simulink model "snb_bc"  (R2012b)
settings: Solver=FixedStepDiscrete  SolverMode=SingleTasking  StartTime=0.0  StopTime=10000  RelTol=1e-3
undefined symbols (not defined in the file): Down, pfb_coeff_gen_calc, Up
libraries: xbsIndex_r4 x19640, casper_library_misc x44, casper_library_delays x18, casper_library_communications x8, xps_library x3
(part 103 of 163)

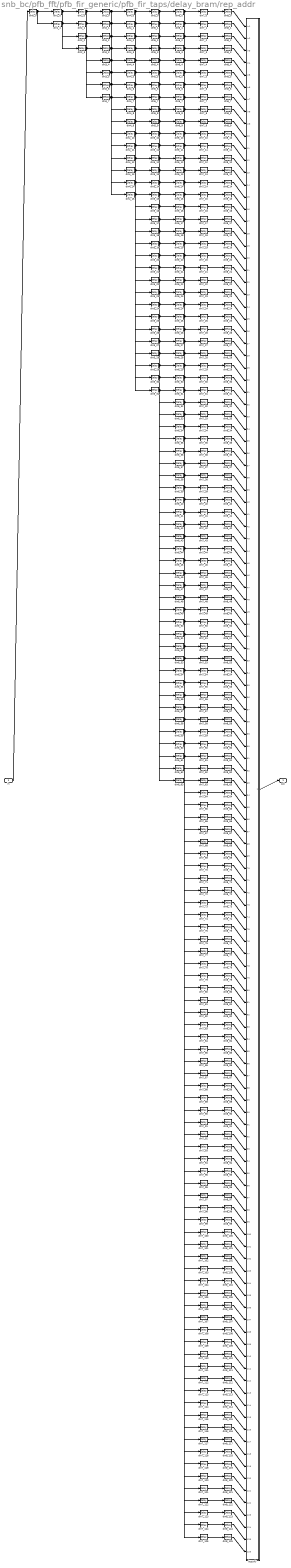
== system snb_bc/pfb_fft/pfb_fir_generic/pfb_fir_taps/delay_bram/rep_addr ==
  in : Inport
  bussify : Subsystem  AncestorBlock=casper_library_flow_control/bus_create  mask(bus_create){inputNum=126}
      mask prompts: inputNum "Number of inputs:"
      mask init:
      | bus_create_init(gcb,...
      |     'inputNum', inputNum);
  din0_0 : xbsIndex_r4/Delay  rst=off  infoeditControl=Selection of Reset will increase slice count due to use of real FFs and instead of SRLs  en=off  latency=1  dbl_ovrd=off  reg_retiming=off  block_type=delay
  din1_0 : xbsIndex_r4/Delay  rst=off  infoeditControl=Selection of Reset will increase slice count due to use of real FFs and instead of SRLs  en=off  latency=1  dbl_ovrd=off  reg_retiming=off  block_type=delay
  din1_1 : xbsIndex_r4/Delay  rst=off  infoeditControl=Selection of Reset will increase slice count due to use of real FFs and instead of SRLs  en=off  latency=1  dbl_ovrd=off  reg_retiming=off  block_type=delay
  din2_{0..3} (4 alike) : xbsIndex_r4/Delay  rst=off  infoeditControl=Selection of Reset will increase slice count due to use of real FFs and instead of SRLs  en=off  latency=1  dbl_ovrd=off  reg_retiming=off  block_type=delay
  din3_{0..7} (8 alike) : xbsIndex_r4/Delay  rst=off  infoeditControl=Selection of Reset will increase slice count due to use of real FFs and instead of SRLs  en=off  latency=1  dbl_ovrd=off  reg_retiming=off  block_type=delay
  din4_{0..15} (16 alike) : xbsIndex_r4/Delay  rst=off  infoeditControl=Selection of Reset will increase slice count due to use of real FFs and instead of SRLs  en=off  latency=1  dbl_ovrd=off  reg_retiming=off  block_type=delay
  din5_{0..31} (32 alike) : xbsIndex_r4/Delay  rst=off  infoeditControl=Selection of Reset will increase slice count due to use of real FFs and instead of SRLs  en=off  latency=1  dbl_ovrd=off  reg_retiming=off  block_type=delay
  din6_{0..63} (64 alike) : xbsIndex_r4/Delay  rst=off  infoeditControl=Selection of Reset will increase slice count due to use of real FFs and instead of SRLs  en=off  latency=1  dbl_ovrd=off  reg_retiming=off  block_type=delay
  din7_{0..125} (126 alike) : xbsIndex_r4/Delay  rst=off  infoeditControl=Selection of Reset will increase slice count due to use of real FFs and instead of SRLs  en=off  latency=1  dbl_ovrd=off  reg_retiming=on  block_type=delay
  din8_{0..125} (126 alike) : xbsIndex_r4/Delay  rst=off  infoeditControl=Selection of Reset will increase slice count due to use of real FFs and instead of SRLs  en=off  latency=1  dbl_ovrd=off  reg_retiming=off  block_type=delay
  out : Outport
  wires:
  bussify/1(bus_out) -> out/1
  din8_125/1 -> bussify/126(in126)
  din8_124/1 -> bussify/125(in125)
  din8_123/1 -> bussify/124(in124)
  din8_122/1 -> bussify/123(in123)
  din8_121/1 -> bussify/122(in122)
  din8_120/1 -> bussify/121(in121)
  din8_119/1 -> bussify/120(in120)
  din8_118/1 -> bussify/119(in119)
  din8_117/1 -> bussify/118(in118)
  din8_116/1 -> bussify/117(in117)
  din8_115/1 -> bussify/116(in116)
  din8_114/1 -> bussify/115(in115)
  din8_113/1 -> bussify/114(in114)
  din8_112/1 -> bussify/113(in113)
  din8_111/1 -> bussify/112(in112)
  din8_110/1 -> bussify/111(in111)
  din8_109/1 -> bussify/110(in110)
  din8_108/1 -> bussify/109(in109)
  din8_107/1 -> bussify/108(in108)
  din8_106/1 -> bussify/107(in107)
  din8_105/1 -> bussify/106(in106)
  din8_104/1 -> bussify/105(in105)
  din8_103/1 -> bussify/104(in104)
  din8_102/1 -> bussify/103(in103)
  din8_101/1 -> bussify/102(in102)
  din8_100/1 -> bussify/101(in101)
  din8_99/1 -> bussify/100(in100)
  din8_98/1 -> bussify/99(in99)
  din8_97/1 -> bussify/98(in98)
  din8_96/1 -> bussify/97(in97)
  din8_95/1 -> bussify/96(in96)
  din8_94/1 -> bussify/95(in95)
  din8_93/1 -> bussify/94(in94)
  din8_92/1 -> bussify/93(in93)
  din8_91/1 -> bussify/92(in92)
  din8_90/1 -> bussify/91(in91)
  din8_89/1 -> bussify/90(in90)
  din8_88/1 -> bussify/89(in89)
  din8_87/1 -> bussify/88(in88)
  din8_86/1 -> bussify/87(in87)
  din8_85/1 -> bussify/86(in86)
  din8_84/1 -> bussify/85(in85)
  din8_83/1 -> bussify/84(in84)
  din8_82/1 -> bussify/83(in83)
  din8_81/1 -> bussify/82(in82)
  din8_80/1 -> bussify/81(in81)
  din8_79/1 -> bussify/80(in80)
  din8_78/1 -> bussify/79(in79)
  din8_77/1 -> bussify/78(in78)
  din8_76/1 -> bussify/77(in77)
  din8_75/1 -> bussify/76(in76)
  din8_74/1 -> bussify/75(in75)
  din8_73/1 -> bussify/74(in74)
  din8_72/1 -> bussify/73(in73)
  din8_71/1 -> bussify/72(in72)
  din8_70/1 -> bussify/71(in71)
  din8_69/1 -> bussify/70(in70)
  din8_68/1 -> bussify/69(in69)
  din8_67/1 -> bussify/68(in68)
  din8_66/1 -> bussify/67(in67)
  din8_65/1 -> bussify/66(in66)
  din8_64/1 -> bussify/65(in65)
  din8_63/1 -> bussify/64(in64)
  din8_62/1 -> bussify/63(in63)
  din8_61/1 -> bussify/62(in62)
  din8_60/1 -> bussify/61(in61)
  din8_59/1 -> bussify/60(in60)
  din8_58/1 -> bussify/59(in59)
  din8_57/1 -> bussify/58(in58)
  din8_56/1 -> bussify/57(in57)
  din8_55/1 -> bussify/56(in56)
  din8_54/1 -> bussify/55(in55)
  din8_53/1 -> bussify/54(in54)
  din8_52/1 -> bussify/53(in53)
  din8_51/1 -> bussify/52(in52)
  din8_50/1 -> bussify/51(in51)
  din8_49/1 -> bussify/50(in50)
  din8_48/1 -> bussify/49(in49)
  din8_47/1 -> bussify/48(in48)
  din8_46/1 -> bussify/47(in47)
  din8_45/1 -> bussify/46(in46)
  din8_44/1 -> bussify/45(in45)
  din8_43/1 -> bussify/44(in44)
  din8_42/1 -> bussify/43(in43)
  din8_41/1 -> bussify/42(in42)
  din8_40/1 -> bussify/41(in41)
  din8_39/1 -> bussify/40(in40)
  din8_38/1 -> bussify/39(in39)
  din8_37/1 -> bussify/38(in38)
  din8_36/1 -> bussify/37(in37)
  din8_35/1 -> bussify/36(in36)
  din8_34/1 -> bussify/35(in35)
  din8_33/1 -> bussify/34(in34)
  din8_32/1 -> bussify/33(in33)
  din8_31/1 -> bussify/32(in32)
  din8_30/1 -> bussify/31(in31)
  din8_29/1 -> bussify/30(in30)
  din8_28/1 -> bussify/29(in29)
  din8_27/1 -> bussify/28(in28)
  din8_26/1 -> bussify/27(in27)
  din8_25/1 -> bussify/26(in26)
  din8_24/1 -> bussify/25(in25)
  din8_23/1 -> bussify/24(in24)
  din8_22/1 -> bussify/23(in23)
  din8_21/1 -> bussify/22(in22)
  din8_20/1 -> bussify/21(in21)
  din8_19/1 -> bussify/20(in20)
  din8_18/1 -> bussify/19(in19)
  din8_17/1 -> bussify/18(in18)
  din8_16/1 -> bussify/17(in17)
  din8_15/1 -> bussify/16(in16)
  din8_14/1 -> bussify/15(in15)
  din8_13/1 -> bussify/14(in14)
  din8_12/1 -> bussify/13(in13)
  din8_11/1 -> bussify/12(in12)
  din8_10/1 -> bussify/11(in11)
  din8_9/1 -> bussify/10(in10)
  din8_8/1 -> bussify/9(in9)
  din8_7/1 -> bussify/8(in8)
  din8_6/1 -> bussify/7(in7)
  din8_5/1 -> bussify/6(in6)
  din8_4/1 -> bussify/5(in5)
  din8_3/1 -> bussify/4(in4)
  din8_2/1 -> bussify/3(in3)
  din8_1/1 -> bussify/2(in2)
  din8_0/1 -> bussify/1(in1)
  din7_125/1 -> din8_125/1
  din7_124/1 -> din8_124/1
  din7_123/1 -> din8_123/1
  din7_122/1 -> din8_122/1
  din7_121/1 -> din8_121/1
  din7_120/1 -> din8_120/1
  din7_119/1 -> din8_119/1
  din7_118/1 -> din8_118/1
  din7_117/1 -> din8_117/1
  din7_116/1 -> din8_116/1
  din7_115/1 -> din8_115/1
  din7_114/1 -> din8_114/1
  din7_113/1 -> din8_113/1
  din7_112/1 -> din8_112/1
  din7_111/1 -> din8_111/1
  din7_110/1 -> din8_110/1
  din7_109/1 -> din8_109/1
  din7_108/1 -> din8_108/1
  din7_107/1 -> din8_107/1
  din7_106/1 -> din8_106/1
  din7_105/1 -> din8_105/1
  din7_104/1 -> din8_104/1
  din7_103/1 -> din8_103/1
  din7_102/1 -> din8_102/1
  din7_101/1 -> din8_101/1
  din7_100/1 -> din8_100/1
  din7_99/1 -> din8_99/1
  din7_98/1 -> din8_98/1
  din7_97/1 -> din8_97/1
  din7_96/1 -> din8_96/1
  din7_95/1 -> din8_95/1
  din7_94/1 -> din8_94/1
  din7_93/1 -> din8_93/1
  din7_92/1 -> din8_92/1
  din7_91/1 -> din8_91/1
  din7_90/1 -> din8_90/1
  din7_89/1 -> din8_89/1
  din7_88/1 -> din8_88/1
  din7_87/1 -> din8_87/1
  din7_86/1 -> din8_86/1
  din7_85/1 -> din8_85/1
  din7_84/1 -> din8_84/1
  din7_83/1 -> din8_83/1
  din7_82/1 -> din8_82/1
  din7_81/1 -> din8_81/1
  din7_80/1 -> din8_80/1
  din7_79/1 -> din8_79/1
  din7_78/1 -> din8_78/1
  din7_77/1 -> din8_77/1
  din7_76/1 -> din8_76/1
  din7_75/1 -> din8_75/1
  din7_74/1 -> din8_74/1
  din7_73/1 -> din8_73/1
  din7_72/1 -> din8_72/1
  din7_71/1 -> din8_71/1
  din7_70/1 -> din8_70/1
  din7_69/1 -> din8_69/1
  din7_68/1 -> din8_68/1
  din7_67/1 -> din8_67/1
  din7_66/1 -> din8_66/1
  din7_65/1 -> din8_65/1
  din7_64/1 -> din8_64/1
  din7_63/1 -> din8_63/1
  din7_62/1 -> din8_62/1
  din7_61/1 -> din8_61/1
  din7_60/1 -> din8_60/1
  din7_59/1 -> din8_59/1
  din7_58/1 -> din8_58/1
  din7_57/1 -> din8_57/1
  din7_56/1 -> din8_56/1
  din7_55/1 -> din8_55/1
  din7_54/1 -> din8_54/1
  din7_53/1 -> din8_53/1
  din7_52/1 -> din8_52/1
  din7_51/1 -> din8_51/1
  din7_50/1 -> din8_50/1
  din7_49/1 -> din8_49/1
  din7_48/1 -> din8_48/1
  din7_47/1 -> din8_47/1
  din7_46/1 -> din8_46/1
  din7_45/1 -> din8_45/1
  din7_44/1 -> din8_44/1
  din7_43/1 -> din8_43/1
  din7_42/1 -> din8_42/1
  din7_41/1 -> din8_41/1
  din7_40/1 -> din8_40/1
  din7_39/1 -> din8_39/1
  din7_38/1 -> din8_38/1
  din7_37/1 -> din8_37/1
  din7_36/1 -> din8_36/1
  din7_35/1 -> din8_35/1
  din7_34/1 -> din8_34/1
  din7_33/1 -> din8_33/1
  din7_32/1 -> din8_32/1
  din7_31/1 -> din8_31/1
  din7_30/1 -> din8_30/1
  din7_29/1 -> din8_29/1
  din7_28/1 -> din8_28/1
  din7_27/1 -> din8_27/1
  din7_26/1 -> din8_26/1
  din7_25/1 -> din8_25/1
  din7_24/1 -> din8_24/1
  din7_23/1 -> din8_23/1
  din7_22/1 -> din8_22/1
  din7_21/1 -> din8_21/1
  din7_20/1 -> din8_20/1
  din7_19/1 -> din8_19/1
  din7_18/1 -> din8_18/1
  din7_17/1 -> din8_17/1
  din7_16/1 -> din8_16/1
  din7_15/1 -> din8_15/1
  din7_14/1 -> din8_14/1
  din7_13/1 -> din8_13/1
  din7_12/1 -> din8_12/1
  din7_11/1 -> din8_11/1
  din7_10/1 -> din8_10/1
  din7_9/1 -> din8_9/1
  din7_8/1 -> din8_8/1
  din7_7/1 -> din8_7/1
  din7_6/1 -> din8_6/1
  din7_5/1 -> din8_5/1
  din7_4/1 -> din8_4/1
  din7_3/1 -> din8_3/1
  din7_2/1 -> din8_2/1
  din7_1/1 -> din8_1/1
  din7_0/1 -> din8_0/1
  din6_63/1 -> din7_63/1
  din6_62/1 -> din7_62/1
  din6_61/1 -> din7_125/1, din7_61/1
  din6_60/1 -> din7_124/1, din7_60/1
  din6_59/1 -> din7_123/1, din7_59/1
  din6_58/1 -> din7_122/1, din7_58/1
  din6_57/1 -> din7_121/1, din7_57/1
  din6_56/1 -> din7_120/1, din7_56/1
  din6_55/1 -> din7_119/1, din7_55/1
  din6_54/1 -> din7_118/1, din7_54/1
  din6_53/1 -> din7_117/1, din7_53/1
  din6_52/1 -> din7_116/1, din7_52/1
  din6_51/1 -> din7_115/1, din7_51/1
  din6_50/1 -> din7_114/1, din7_50/1
  din6_49/1 -> din7_113/1, din7_49/1
  din6_48/1 -> din7_112/1, din7_48/1
  din6_47/1 -> din7_111/1, din7_47/1
  din6_46/1 -> din7_110/1, din7_46/1
  din6_45/1 -> din7_109/1, din7_45/1
  din6_44/1 -> din7_108/1, din7_44/1
  din6_43/1 -> din7_107/1, din7_43/1
  din6_42/1 -> din7_106/1, din7_42/1
  din6_41/1 -> din7_105/1, din7_41/1
  din6_40/1 -> din7_104/1, din7_40/1
  din6_39/1 -> din7_103/1, din7_39/1
  din6_38/1 -> din7_102/1, din7_38/1
  din6_37/1 -> din7_101/1, din7_37/1
  din6_36/1 -> din7_100/1, din7_36/1
  din6_35/1 -> din7_99/1, din7_35/1
  din6_34/1 -> din7_98/1, din7_34/1
  din6_33/1 -> din7_97/1, din7_33/1
  din6_32/1 -> din7_96/1, din7_32/1
  din6_31/1 -> din7_95/1, din7_31/1
  din6_30/1 -> din7_94/1, din7_30/1
  din6_29/1 -> din7_93/1, din7_29/1
  din6_28/1 -> din7_92/1, din7_28/1
  din6_27/1 -> din7_91/1, din7_27/1
  din6_26/1 -> din7_90/1, din7_26/1
  din6_25/1 -> din7_89/1, din7_25/1
  din6_24/1 -> din7_88/1, din7_24/1
  din6_23/1 -> din7_87/1, din7_23/1
  din6_22/1 -> din7_86/1, din7_22/1
  din6_21/1 -> din7_85/1, din7_21/1
  din6_20/1 -> din7_84/1, din7_20/1
  din6_19/1 -> din7_83/1, din7_19/1
  din6_18/1 -> din7_82/1, din7_18/1
  din6_17/1 -> din7_81/1, din7_17/1
  din6_16/1 -> din7_80/1, din7_16/1
  din6_15/1 -> din7_79/1, din7_15/1
  din6_14/1 -> din7_78/1, din7_14/1
  din6_13/1 -> din7_77/1, din7_13/1
  din6_12/1 -> din7_76/1, din7_12/1
  din6_11/1 -> din7_75/1, din7_11/1
  din6_10/1 -> din7_74/1, din7_10/1
  din6_9/1 -> din7_73/1, din7_9/1
  din6_8/1 -> din7_72/1, din7_8/1
  din6_7/1 -> din7_71/1, din7_7/1
  din6_6/1 -> din7_70/1, din7_6/1
  din6_5/1 -> din7_69/1, din7_5/1
  din6_4/1 -> din7_68/1, din7_4/1
  din6_3/1 -> din7_67/1, din7_3/1
  din6_2/1 -> din7_66/1, din7_2/1
  din6_1/1 -> din7_65/1, din7_1/1
  din6_0/1 -> din7_64/1, din7_0/1
  din5_31/1 -> din6_63/1, din6_31/1
  din5_30/1 -> din6_62/1, din6_30/1
  din5_29/1 -> din6_61/1, din6_29/1
  din5_28/1 -> din6_60/1, din6_28/1
  din5_27/1 -> din6_59/1, din6_27/1
  din5_26/1 -> din6_58/1, din6_26/1
  din5_25/1 -> din6_57/1, din6_25/1
  din5_24/1 -> din6_56/1, din6_24/1
  din5_23/1 -> din6_55/1, din6_23/1
  din5_22/1 -> din6_54/1, din6_22/1
  din5_21/1 -> din6_53/1, din6_21/1
  din5_20/1 -> din6_52/1, din6_20/1
  din5_19/1 -> din6_51/1, din6_19/1
  din5_18/1 -> din6_50/1, din6_18/1
  din5_17/1 -> din6_49/1, din6_17/1
  din5_16/1 -> din6_48/1, din6_16/1
  din5_15/1 -> din6_47/1, din6_15/1
  din5_14/1 -> din6_46/1, din6_14/1
  din5_13/1 -> din6_45/1, din6_13/1
  din5_12/1 -> din6_44/1, din6_12/1
  din5_11/1 -> din6_43/1, din6_11/1
  din5_10/1 -> din6_42/1, din6_10/1
  din5_9/1 -> din6_41/1, din6_9/1
  din5_8/1 -> din6_40/1, din6_8/1
  din5_7/1 -> din6_39/1, din6_7/1
  din5_6/1 -> din6_38/1, din6_6/1
  din5_5/1 -> din6_37/1, din6_5/1
  din5_4/1 -> din6_36/1, din6_4/1
  din5_3/1 -> din6_35/1, din6_3/1
  din5_2/1 -> din6_34/1, din6_2/1
  din5_1/1 -> din6_33/1, din6_1/1
  din5_0/1 -> din6_32/1, din6_0/1
  din4_15/1 -> din5_31/1, din5_15/1
  din4_14/1 -> din5_30/1, din5_14/1
  din4_13/1 -> din5_29/1, din5_13/1
  din4_12/1 -> din5_28/1, din5_12/1
  din4_11/1 -> din5_27/1, din5_11/1
  din4_10/1 -> din5_26/1, din5_10/1
  din4_9/1 -> din5_25/1, din5_9/1
  din4_8/1 -> din5_24/1, din5_8/1
  din4_7/1 -> din5_23/1, din5_7/1
  din4_6/1 -> din5_22/1, din5_6/1
  din4_5/1 -> din5_21/1, din5_5/1
  din4_4/1 -> din5_20/1, din5_4/1
  din4_3/1 -> din5_19/1, din5_3/1
  din4_2/1 -> din5_18/1, din5_2/1
  din4_1/1 -> din5_17/1, din5_1/1
  din4_0/1 -> din5_16/1, din5_0/1
  din3_7/1 -> din4_15/1, din4_7/1
  din3_6/1 -> din4_14/1, din4_6/1
  din3_5/1 -> din4_13/1, din4_5/1
  din3_4/1 -> din4_12/1, din4_4/1
  din3_3/1 -> din4_11/1, din4_3/1
  din3_2/1 -> din4_10/1, din4_2/1
  din3_1/1 -> din4_9/1, din4_1/1
  din3_0/1 -> din4_8/1, din4_0/1
  din2_3/1 -> din3_7/1, din3_3/1
  din2_2/1 -> din3_6/1, din3_2/1
  din2_1/1 -> din3_5/1, din3_1/1
  din2_0/1 -> din3_4/1, din3_0/1
  din1_1/1 -> din2_3/1, din2_1/1
  din1_0/1 -> din2_2/1, din2_0/1
  din0_0/1 -> din1_1/1, din1_0/1
  in/1 -> din0_0/1

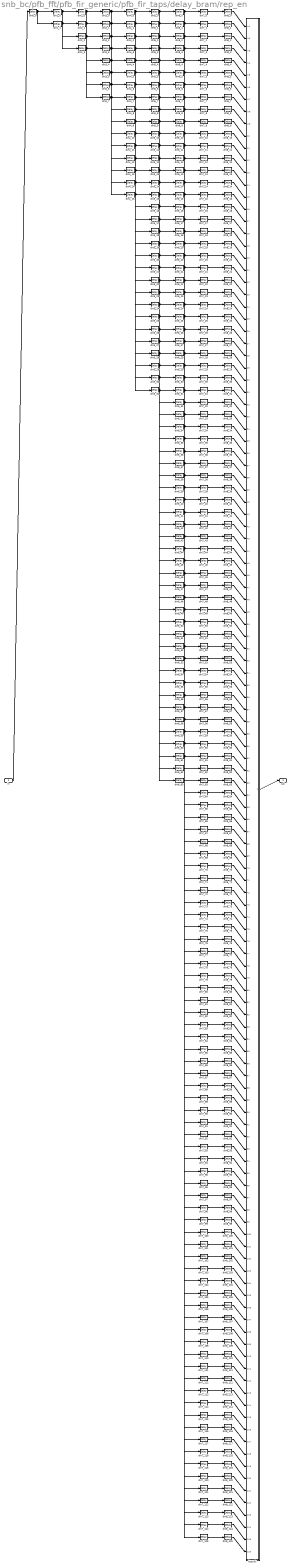
== system snb_bc/pfb_fft/pfb_fir_generic/pfb_fir_taps/delay_bram/rep_en ==
  in : Inport
  bussify : Subsystem  AncestorBlock=casper_library_flow_control/bus_create  mask(bus_create){inputNum=126}
      mask prompts: inputNum "Number of inputs:"
      mask init:
      | bus_create_init(gcb,...
      |     'inputNum', inputNum);
  din0_0 : xbsIndex_r4/Delay  rst=off  infoeditControl=Selection of Reset will increase slice count due to use of real FFs and instead of SRLs  en=off  latency=1  dbl_ovrd=off  reg_retiming=off  block_type=delay
  din1_0 : xbsIndex_r4/Delay  rst=off  infoeditControl=Selection of Reset will increase slice count due to use of real FFs and instead of SRLs  en=off  latency=1  dbl_ovrd=off  reg_retiming=off  block_type=delay
  din1_1 : xbsIndex_r4/Delay  rst=off  infoeditControl=Selection of Reset will increase slice count due to use of real FFs and instead of SRLs  en=off  latency=1  dbl_ovrd=off  reg_retiming=off  block_type=delay
  din2_{0..3} (4 alike) : xbsIndex_r4/Delay  rst=off  infoeditControl=Selection of Reset will increase slice count due to use of real FFs and instead of SRLs  en=off  latency=1  dbl_ovrd=off  reg_retiming=off  block_type=delay
  din3_{0..7} (8 alike) : xbsIndex_r4/Delay  rst=off  infoeditControl=Selection of Reset will increase slice count due to use of real FFs and instead of SRLs  en=off  latency=1  dbl_ovrd=off  reg_retiming=off  block_type=delay
  din4_{0..15} (16 alike) : xbsIndex_r4/Delay  rst=off  infoeditControl=Selection of Reset will increase slice count due to use of real FFs and instead of SRLs  en=off  latency=1  dbl_ovrd=off  reg_retiming=off  block_type=delay
  din5_{0..31} (32 alike) : xbsIndex_r4/Delay  rst=off  infoeditControl=Selection of Reset will increase slice count due to use of real FFs and instead of SRLs  en=off  latency=1  dbl_ovrd=off  reg_retiming=off  block_type=delay
  din6_{0..63} (64 alike) : xbsIndex_r4/Delay  rst=off  infoeditControl=Selection of Reset will increase slice count due to use of real FFs and instead of SRLs  en=off  latency=1  dbl_ovrd=off  reg_retiming=off  block_type=delay
  din7_{0..125} (126 alike) : xbsIndex_r4/Delay  rst=off  infoeditControl=Selection of Reset will increase slice count due to use of real FFs and instead of SRLs  en=off  latency=1  dbl_ovrd=off  reg_retiming=on  block_type=delay
  din8_{0..125} (126 alike) : xbsIndex_r4/Delay  rst=off  infoeditControl=Selection of Reset will increase slice count due to use of real FFs and instead of SRLs  en=off  latency=1  dbl_ovrd=off  reg_retiming=off  block_type=delay
  out : Outport
  wires:
  bussify/1(bus_out) -> out/1
  din8_125/1 -> bussify/126(in126)
  din8_124/1 -> bussify/125(in125)
  din8_123/1 -> bussify/124(in124)
  din8_122/1 -> bussify/123(in123)
  din8_121/1 -> bussify/122(in122)
  din8_120/1 -> bussify/121(in121)
  din8_119/1 -> bussify/120(in120)
  din8_118/1 -> bussify/119(in119)
  din8_117/1 -> bussify/118(in118)
  din8_116/1 -> bussify/117(in117)
  din8_115/1 -> bussify/116(in116)
  din8_114/1 -> bussify/115(in115)
  din8_113/1 -> bussify/114(in114)
  din8_112/1 -> bussify/113(in113)
  din8_111/1 -> bussify/112(in112)
  din8_110/1 -> bussify/111(in111)
  din8_109/1 -> bussify/110(in110)
  din8_108/1 -> bussify/109(in109)
  din8_107/1 -> bussify/108(in108)
  din8_106/1 -> bussify/107(in107)
  din8_105/1 -> bussify/106(in106)
  din8_104/1 -> bussify/105(in105)
  din8_103/1 -> bussify/104(in104)
  din8_102/1 -> bussify/103(in103)
  din8_101/1 -> bussify/102(in102)
  din8_100/1 -> bussify/101(in101)
  din8_99/1 -> bussify/100(in100)
  din8_98/1 -> bussify/99(in99)
  din8_97/1 -> bussify/98(in98)
  din8_96/1 -> bussify/97(in97)
  din8_95/1 -> bussify/96(in96)
  din8_94/1 -> bussify/95(in95)
  din8_93/1 -> bussify/94(in94)
  din8_92/1 -> bussify/93(in93)
  din8_91/1 -> bussify/92(in92)
  din8_90/1 -> bussify/91(in91)
  din8_89/1 -> bussify/90(in90)
  din8_88/1 -> bussify/89(in89)
  din8_87/1 -> bussify/88(in88)
  din8_86/1 -> bussify/87(in87)
  din8_85/1 -> bussify/86(in86)
  din8_84/1 -> bussify/85(in85)
  din8_83/1 -> bussify/84(in84)
  din8_82/1 -> bussify/83(in83)
  din8_81/1 -> bussify/82(in82)
  din8_80/1 -> bussify/81(in81)
  din8_79/1 -> bussify/80(in80)
  din8_78/1 -> bussify/79(in79)
  din8_77/1 -> bussify/78(in78)
  din8_76/1 -> bussify/77(in77)
  din8_75/1 -> bussify/76(in76)
  din8_74/1 -> bussify/75(in75)
  din8_73/1 -> bussify/74(in74)
  din8_72/1 -> bussify/73(in73)
  din8_71/1 -> bussify/72(in72)
  din8_70/1 -> bussify/71(in71)
  din8_69/1 -> bussify/70(in70)
  din8_68/1 -> bussify/69(in69)
  din8_67/1 -> bussify/68(in68)
  din8_66/1 -> bussify/67(in67)
  din8_65/1 -> bussify/66(in66)
  din8_64/1 -> bussify/65(in65)
  din8_63/1 -> bussify/64(in64)
  din8_62/1 -> bussify/63(in63)
  din8_61/1 -> bussify/62(in62)
  din8_60/1 -> bussify/61(in61)
  din8_59/1 -> bussify/60(in60)
  din8_58/1 -> bussify/59(in59)
  din8_57/1 -> bussify/58(in58)
  din8_56/1 -> bussify/57(in57)
  din8_55/1 -> bussify/56(in56)
  din8_54/1 -> bussify/55(in55)
  din8_53/1 -> bussify/54(in54)
  din8_52/1 -> bussify/53(in53)
  din8_51/1 -> bussify/52(in52)
  din8_50/1 -> bussify/51(in51)
  din8_49/1 -> bussify/50(in50)
  din8_48/1 -> bussify/49(in49)
  din8_47/1 -> bussify/48(in48)
  din8_46/1 -> bussify/47(in47)
  din8_45/1 -> bussify/46(in46)
  din8_44/1 -> bussify/45(in45)
  din8_43/1 -> bussify/44(in44)
  din8_42/1 -> bussify/43(in43)
  din8_41/1 -> bussify/42(in42)
  din8_40/1 -> bussify/41(in41)
  din8_39/1 -> bussify/40(in40)
  din8_38/1 -> bussify/39(in39)
  din8_37/1 -> bussify/38(in38)
  din8_36/1 -> bussify/37(in37)
  din8_35/1 -> bussify/36(in36)
  din8_34/1 -> bussify/35(in35)
  din8_33/1 -> bussify/34(in34)
  din8_32/1 -> bussify/33(in33)
  din8_31/1 -> bussify/32(in32)
  din8_30/1 -> bussify/31(in31)
  din8_29/1 -> bussify/30(in30)
  din8_28/1 -> bussify/29(in29)
  din8_27/1 -> bussify/28(in28)
  din8_26/1 -> bussify/27(in27)
  din8_25/1 -> bussify/26(in26)
  din8_24/1 -> bussify/25(in25)
  din8_23/1 -> bussify/24(in24)
  din8_22/1 -> bussify/23(in23)
  din8_21/1 -> bussify/22(in22)
  din8_20/1 -> bussify/21(in21)
  din8_19/1 -> bussify/20(in20)
  din8_18/1 -> bussify/19(in19)
  din8_17/1 -> bussify/18(in18)
  din8_16/1 -> bussify/17(in17)
  din8_15/1 -> bussify/16(in16)
  din8_14/1 -> bussify/15(in15)
  din8_13/1 -> bussify/14(in14)
  din8_12/1 -> bussify/13(in13)
  din8_11/1 -> bussify/12(in12)
  din8_10/1 -> bussify/11(in11)
  din8_9/1 -> bussify/10(in10)
  din8_8/1 -> bussify/9(in9)
  din8_7/1 -> bussify/8(in8)
  din8_6/1 -> bussify/7(in7)
  din8_5/1 -> bussify/6(in6)
  din8_4/1 -> bussify/5(in5)
  din8_3/1 -> bussify/4(in4)
  din8_2/1 -> bussify/3(in3)
  din8_1/1 -> bussify/2(in2)
  din8_0/1 -> bussify/1(in1)
  din7_125/1 -> din8_125/1
  din7_124/1 -> din8_124/1
  din7_123/1 -> din8_123/1
  din7_122/1 -> din8_122/1
  din7_121/1 -> din8_121/1
  din7_120/1 -> din8_120/1
  din7_119/1 -> din8_119/1
  din7_118/1 -> din8_118/1
  din7_117/1 -> din8_117/1
  din7_116/1 -> din8_116/1
  din7_115/1 -> din8_115/1
  din7_114/1 -> din8_114/1
  din7_113/1 -> din8_113/1
  din7_112/1 -> din8_112/1
  din7_111/1 -> din8_111/1
  din7_110/1 -> din8_110/1
  din7_109/1 -> din8_109/1
  din7_108/1 -> din8_108/1
  din7_107/1 -> din8_107/1
  din7_106/1 -> din8_106/1
  din7_105/1 -> din8_105/1
  din7_104/1 -> din8_104/1
  din7_103/1 -> din8_103/1
  din7_102/1 -> din8_102/1
  din7_101/1 -> din8_101/1
  din7_100/1 -> din8_100/1
  din7_99/1 -> din8_99/1
  din7_98/1 -> din8_98/1
  din7_97/1 -> din8_97/1
  din7_96/1 -> din8_96/1
  din7_95/1 -> din8_95/1
  din7_94/1 -> din8_94/1
  din7_93/1 -> din8_93/1
  din7_92/1 -> din8_92/1
  din7_91/1 -> din8_91/1
  din7_90/1 -> din8_90/1
  din7_89/1 -> din8_89/1
  din7_88/1 -> din8_88/1
  din7_87/1 -> din8_87/1
  din7_86/1 -> din8_86/1
  din7_85/1 -> din8_85/1
  din7_84/1 -> din8_84/1
  din7_83/1 -> din8_83/1
  din7_82/1 -> din8_82/1
  din7_81/1 -> din8_81/1
  din7_80/1 -> din8_80/1
  din7_79/1 -> din8_79/1
  din7_78/1 -> din8_78/1
  din7_77/1 -> din8_77/1
  din7_76/1 -> din8_76/1
  din7_75/1 -> din8_75/1
  din7_74/1 -> din8_74/1
  din7_73/1 -> din8_73/1
  din7_72/1 -> din8_72/1
  din7_71/1 -> din8_71/1
  din7_70/1 -> din8_70/1
  din7_69/1 -> din8_69/1
  din7_68/1 -> din8_68/1
  din7_67/1 -> din8_67/1
  din7_66/1 -> din8_66/1
  din7_65/1 -> din8_65/1
  din7_64/1 -> din8_64/1
  din7_63/1 -> din8_63/1
  din7_62/1 -> din8_62/1
  din7_61/1 -> din8_61/1
  din7_60/1 -> din8_60/1
  din7_59/1 -> din8_59/1
  din7_58/1 -> din8_58/1
  din7_57/1 -> din8_57/1
  din7_56/1 -> din8_56/1
  din7_55/1 -> din8_55/1
  din7_54/1 -> din8_54/1
  din7_53/1 -> din8_53/1
  din7_52/1 -> din8_52/1
  din7_51/1 -> din8_51/1
  din7_50/1 -> din8_50/1
  din7_49/1 -> din8_49/1
  din7_48/1 -> din8_48/1
  din7_47/1 -> din8_47/1
  din7_46/1 -> din8_46/1
  din7_45/1 -> din8_45/1
  din7_44/1 -> din8_44/1
  din7_43/1 -> din8_43/1
  din7_42/1 -> din8_42/1
  din7_41/1 -> din8_41/1
  din7_40/1 -> din8_40/1
  din7_39/1 -> din8_39/1
  din7_38/1 -> din8_38/1
  din7_37/1 -> din8_37/1
  din7_36/1 -> din8_36/1
  din7_35/1 -> din8_35/1
  din7_34/1 -> din8_34/1
  din7_33/1 -> din8_33/1
  din7_32/1 -> din8_32/1
  din7_31/1 -> din8_31/1
  din7_30/1 -> din8_30/1
  din7_29/1 -> din8_29/1
  din7_28/1 -> din8_28/1
  din7_27/1 -> din8_27/1
  din7_26/1 -> din8_26/1
  din7_25/1 -> din8_25/1
  din7_24/1 -> din8_24/1
  din7_23/1 -> din8_23/1
  din7_22/1 -> din8_22/1
  din7_21/1 -> din8_21/1
  din7_20/1 -> din8_20/1
  din7_19/1 -> din8_19/1
  din7_18/1 -> din8_18/1
  din7_17/1 -> din8_17/1
  din7_16/1 -> din8_16/1
  din7_15/1 -> din8_15/1
  din7_14/1 -> din8_14/1
  din7_13/1 -> din8_13/1
  din7_12/1 -> din8_12/1
  din7_11/1 -> din8_11/1
  din7_10/1 -> din8_10/1
  din7_9/1 -> din8_9/1
  din7_8/1 -> din8_8/1
  din7_7/1 -> din8_7/1
  din7_6/1 -> din8_6/1
  din7_5/1 -> din8_5/1
  din7_4/1 -> din8_4/1
  din7_3/1 -> din8_3/1
  din7_2/1 -> din8_2/1
  din7_1/1 -> din8_1/1
  din7_0/1 -> din8_0/1
  din6_63/1 -> din7_63/1
  din6_62/1 -> din7_62/1
  din6_61/1 -> din7_125/1, din7_61/1
  din6_60/1 -> din7_124/1, din7_60/1
  din6_59/1 -> din7_123/1, din7_59/1
  din6_58/1 -> din7_122/1, din7_58/1
  din6_57/1 -> din7_121/1, din7_57/1
  din6_56/1 -> din7_120/1, din7_56/1
  din6_55/1 -> din7_119/1, din7_55/1
  din6_54/1 -> din7_118/1, din7_54/1
  din6_53/1 -> din7_117/1, din7_53/1
  din6_52/1 -> din7_116/1, din7_52/1
  din6_51/1 -> din7_115/1, din7_51/1
  din6_50/1 -> din7_114/1, din7_50/1
  din6_49/1 -> din7_113/1, din7_49/1
  din6_48/1 -> din7_112/1, din7_48/1
  din6_47/1 -> din7_111/1, din7_47/1
  din6_46/1 -> din7_110/1, din7_46/1
  din6_45/1 -> din7_109/1, din7_45/1
  din6_44/1 -> din7_108/1, din7_44/1
  din6_43/1 -> din7_107/1, din7_43/1
  din6_42/1 -> din7_106/1, din7_42/1
  din6_41/1 -> din7_105/1, din7_41/1
  din6_40/1 -> din7_104/1, din7_40/1
  din6_39/1 -> din7_103/1, din7_39/1
  din6_38/1 -> din7_102/1, din7_38/1
  din6_37/1 -> din7_101/1, din7_37/1
  din6_36/1 -> din7_100/1, din7_36/1
  din6_35/1 -> din7_99/1, din7_35/1
  din6_34/1 -> din7_98/1, din7_34/1
  din6_33/1 -> din7_97/1, din7_33/1
  din6_32/1 -> din7_96/1, din7_32/1
  din6_31/1 -> din7_95/1, din7_31/1
  din6_30/1 -> din7_94/1, din7_30/1
  din6_29/1 -> din7_93/1, din7_29/1
  din6_28/1 -> din7_92/1, din7_28/1
  din6_27/1 -> din7_91/1, din7_27/1
  din6_26/1 -> din7_90/1, din7_26/1
  din6_25/1 -> din7_89/1, din7_25/1
  din6_24/1 -> din7_88/1, din7_24/1
  din6_23/1 -> din7_87/1, din7_23/1
  din6_22/1 -> din7_86/1, din7_22/1
  din6_21/1 -> din7_85/1, din7_21/1
  din6_20/1 -> din7_84/1, din7_20/1
  din6_19/1 -> din7_83/1, din7_19/1
  din6_18/1 -> din7_82/1, din7_18/1
  din6_17/1 -> din7_81/1, din7_17/1
  din6_16/1 -> din7_80/1, din7_16/1
  din6_15/1 -> din7_79/1, din7_15/1
  din6_14/1 -> din7_78/1, din7_14/1
  din6_13/1 -> din7_77/1, din7_13/1
  din6_12/1 -> din7_76/1, din7_12/1
  din6_11/1 -> din7_75/1, din7_11/1
  din6_10/1 -> din7_74/1, din7_10/1
  din6_9/1 -> din7_73/1, din7_9/1
  din6_8/1 -> din7_72/1, din7_8/1
  din6_7/1 -> din7_71/1, din7_7/1
  din6_6/1 -> din7_70/1, din7_6/1
  din6_5/1 -> din7_69/1, din7_5/1
  din6_4/1 -> din7_68/1, din7_4/1
  din6_3/1 -> din7_67/1, din7_3/1
  din6_2/1 -> din7_66/1, din7_2/1
  din6_1/1 -> din7_65/1, din7_1/1
  din6_0/1 -> din7_64/1, din7_0/1
  din5_31/1 -> din6_63/1, din6_31/1
  din5_30/1 -> din6_62/1, din6_30/1
  din5_29/1 -> din6_61/1, din6_29/1
  din5_28/1 -> din6_60/1, din6_28/1
  din5_27/1 -> din6_59/1, din6_27/1
  din5_26/1 -> din6_58/1, din6_26/1
  din5_25/1 -> din6_57/1, din6_25/1
  din5_24/1 -> din6_56/1, din6_24/1
  din5_23/1 -> din6_55/1, din6_23/1
  din5_22/1 -> din6_54/1, din6_22/1
  din5_21/1 -> din6_53/1, din6_21/1
  din5_20/1 -> din6_52/1, din6_20/1
  din5_19/1 -> din6_51/1, din6_19/1
  din5_18/1 -> din6_50/1, din6_18/1
  din5_17/1 -> din6_49/1, din6_17/1
  din5_16/1 -> din6_48/1, din6_16/1
  din5_15/1 -> din6_47/1, din6_15/1
  din5_14/1 -> din6_46/1, din6_14/1
  din5_13/1 -> din6_45/1, din6_13/1
  din5_12/1 -> din6_44/1, din6_12/1
  din5_11/1 -> din6_43/1, din6_11/1
  din5_10/1 -> din6_42/1, din6_10/1
  din5_9/1 -> din6_41/1, din6_9/1
  din5_8/1 -> din6_40/1, din6_8/1
  din5_7/1 -> din6_39/1, din6_7/1
  din5_6/1 -> din6_38/1, din6_6/1
  din5_5/1 -> din6_37/1, din6_5/1
  din5_4/1 -> din6_36/1, din6_4/1
  din5_3/1 -> din6_35/1, din6_3/1
  din5_2/1 -> din6_34/1, din6_2/1
  din5_1/1 -> din6_33/1, din6_1/1
  din5_0/1 -> din6_32/1, din6_0/1
  din4_15/1 -> din5_31/1, din5_15/1
  din4_14/1 -> din5_30/1, din5_14/1
  din4_13/1 -> din5_29/1, din5_13/1
  din4_12/1 -> din5_28/1, din5_12/1
  din4_11/1 -> din5_27/1, din5_11/1
  din4_10/1 -> din5_26/1, din5_10/1
  din4_9/1 -> din5_25/1, din5_9/1
  din4_8/1 -> din5_24/1, din5_8/1
  din4_7/1 -> din5_23/1, din5_7/1
  din4_6/1 -> din5_22/1, din5_6/1
  din4_5/1 -> din5_21/1, din5_5/1
  din4_4/1 -> din5_20/1, din5_4/1
  din4_3/1 -> din5_19/1, din5_3/1
  din4_2/1 -> din5_18/1, din5_2/1
  din4_1/1 -> din5_17/1, din5_1/1
  din4_0/1 -> din5_16/1, din5_0/1
  din3_7/1 -> din4_15/1, din4_7/1
  din3_6/1 -> din4_14/1, din4_6/1
  din3_5/1 -> din4_13/1, din4_5/1
  din3_4/1 -> din4_12/1, din4_4/1
  din3_3/1 -> din4_11/1, din4_3/1
  din3_2/1 -> din4_10/1, din4_2/1
  din3_1/1 -> din4_9/1, din4_1/1
  din3_0/1 -> din4_8/1, din4_0/1
  din2_3/1 -> din3_7/1, din3_3/1
  din2_2/1 -> din3_6/1, din3_2/1
  din2_1/1 -> din3_5/1, din3_1/1
  din2_0/1 -> din3_4/1, din3_0/1
  din1_1/1 -> din2_3/1, din2_1/1
  din1_0/1 -> din2_2/1, din2_0/1
  din0_0/1 -> din1_1/1, din1_0/1
  in/1 -> din0_0/1

== system snb_bc/pfb_fft/pfb_fir_generic/pfb_fir_taps/delay_bram/rep_we ==
  in : Inport
  bussify : Subsystem  AncestorBlock=casper_library_flow_control/bus_create  mask(bus_create){inputNum=126}
      mask prompts: inputNum "Number of inputs:"
      mask init:
      | bus_create_init(gcb,...
      |     'inputNum', inputNum);
  out : Outport
  wires:
  bussify/1(bus_out) -> out/1
  in/1 -> bussify/126(in126), bussify/125(in125), bussify/124(in124), bussify/123(in123), bussify/122(in122), bussify/121(in121), bussify/120(in120), bussify/119(in119), bussify/118(in118), bussify/117(in117), bussify/116(in116), bussify/115(in115), bussify/114(in114), bussify/113(in113), bussify/112(in112), bussify/111(in111), bussify/110(in110), bussify/109(in109), bussify/108(in108), bussify/107(in107), bussify/106(in106), bussify/105(in105), bussify/104(in104), bussify/103(in103), bussify/102(in102), bussify/101(in101), bussify/100(in100), bussify/99(in99), bussify/98(in98), bussify/97(in97), bussify/96(in96), bussify/95(in95), bussify/94(in94), bussify/93(in93), bussify/92(in92), bussify/91(in91), bussify/90(in90), bussify/89(in89), bussify/88(in88), bussify/87(in87), bussify/86(in86), bussify/85(in85), bussify/84(in84), bussify/83(in83), bussify/82(in82), bussify/81(in81), bussify/80(in80), bussify/79(in79), bussify/78(in78), bussify/77(in77), bussify/76(in76), bussify/75(in75), bussify/74(in74), bussify/73(in73), bussify/72(in72), bussify/71(in71), bussify/70(in70), bussify/69(in69), bussify/68(in68), bussify/67(in67), bussify/66(in66), bussify/65(in65), bussify/64(in64), bussify/63(in63), bussify/62(in62), bussify/61(in61), bussify/60(in60), bussify/59(in59), bussify/58(in58), bussify/57(in57), bussify/56(in56), bussify/55(in55), bussify/54(in54), bussify/53(in53), bussify/52(in52), bussify/51(in51), bussify/50(in50), bussify/49(in49), bussify/48(in48), bussify/47(in47), bussify/46(in46), bussify/45(in45), bussify/44(in44), bussify/43(in43), bussify/42(in42), bussify/41(in41), bussify/40(in40), bussify/39(in39), bussify/38(in38), bussify/37(in37), bussify/36(in36), bussify/35(in35), bussify/34(in34), bussify/33(in33), bussify/32(in32), bussify/31(in31), bussify/30(in30), bussify/29(in29), bussify/28(in28), bussify/27(in27), bussify/26(in26), bussify/25(in25), bussify/24(in24), bussify/23(in23), bussify/22(in22), bussify/21(in21), bussify/20(in20), bussify/19(in19), bussify/18(in18), bussify/17(in17), bussify/16(in16), bussify/15(in15), bussify/14(in14), bussify/13(in13), bussify/12(in12), bussify/11(in11), bussify/10(in10), bussify/9(in9), bussify/8(in8), bussify/7(in7), bussify/6(in6), bussify/5(in5), bussify/4(in4), bussify/3(in3), bussify/2(in2), bussify/1(in1)

== system snb_bc/pfb_fft/pfb_fir_generic/pfb_fir_taps/en_replicate0/bussify ==
  in1 : Inport
  in2 : Inport  Port=2
  in3 : Inport  Port=3
  in4 : Inport  Port=4
  in5 : Inport  Port=5
  in6 : Inport  Port=6
  in7 : Inport  Port=7
  in8 : Inport  Port=8
  in9 : Inport  Port=9
  in10 : Inport  Port=10
  in11 : Inport  Port=11
  in12 : Inport  Port=12
  in13 : Inport  Port=13
  in14 : Inport  Port=14
  concatenate : xbsIndex_r4/Concat  num_inputs=14  dbl_ovrd=off  block_type=concat
  reinterpret{1..14} (14 alike) : xbsIndex_r4/Reinterpret  force_arith_type=on  arith_type=Unsigned  force_bin_pt=on  bin_pt=0  block_type=reinterpret
      reinterpret1 settings: infoedit="Changes signal type without altering the binary representation.   You can changed the signal between signed and unsigned, and relocate the binary point.<br><br>Hardware notes: In hardware this block costs nothing.<br><br>Example:  Suppose the input is 6 bits wide, signed, with 2 fractional bits, and the output is forced to unsigned with 0 fractional bits.  Then an input of -2.0 (1110.00 in binary 2's complement) becomes an output of 56 (111000 in binary)."
      reinterpret2 settings: infoedit="Changes signal type without altering the binary representation.   You can changed the signal between signed and unsigned, and relocate the binary point.<br><br>Hardware notes: In hardware this block costs nothing.<br><br>Example:  Suppose the input is 6 bits wide, signed, with 2 fractional bits, and the output is forced to unsigned with 0 fractional bits.  Then an input of -2.0 (1110.00 in binary 2's complement) becomes an output of 56 (111000 in binary)."
  bus_out : Outport
  wires:
  reinterpret14/1 -> concatenate/14
  in14/1 -> reinterpret14/1
  reinterpret13/1 -> concatenate/13
  in13/1 -> reinterpret13/1
  reinterpret12/1 -> concatenate/12
  in12/1 -> reinterpret12/1
  reinterpret11/1 -> concatenate/11
  in11/1 -> reinterpret11/1
  reinterpret10/1 -> concatenate/10
  in10/1 -> reinterpret10/1
  reinterpret9/1 -> concatenate/9
  in9/1 -> reinterpret9/1
  reinterpret8/1 -> concatenate/8
  in8/1 -> reinterpret8/1
  reinterpret7/1 -> concatenate/7
  in7/1 -> reinterpret7/1
  reinterpret6/1 -> concatenate/6
  in6/1 -> reinterpret6/1
  reinterpret5/1 -> concatenate/5
  in5/1 -> reinterpret5/1
  reinterpret4/1 -> concatenate/4
  in4/1 -> reinterpret4/1
  reinterpret3/1 -> concatenate/3
  in3/1 -> reinterpret3/1
  reinterpret2/1 -> concatenate/2
  in2/1 -> reinterpret2/1
  reinterpret1/1 -> concatenate/1
  in1/1 -> reinterpret1/1
  concatenate/1 -> bus_out/1

== system snb_bc/pfb_fft/pfb_fir_generic/pfb_fir_taps/en_replicate1/bussify ==
  in1 : Inport
  in2 : Inport  Port=2
  in3 : Inport  Port=3
  in4 : Inport  Port=4
  in5 : Inport  Port=5
  in6 : Inport  Port=6
  in7 : Inport  Port=7
  in8 : Inport  Port=8
  in9 : Inport  Port=9
  in10 : Inport  Port=10
  in11 : Inport  Port=11
  in12 : Inport  Port=12
  in13 : Inport  Port=13
  in14 : Inport  Port=14
  in15 : Inport  Port=15
  in16 : Inport  Port=16
  concatenate : xbsIndex_r4/Concat  num_inputs=16  dbl_ovrd=off  block_type=concat
  reinterpret{1..16} (16 alike) : xbsIndex_r4/Reinterpret  force_arith_type=on  arith_type=Unsigned  force_bin_pt=on  bin_pt=0  block_type=reinterpret
      reinterpret1 settings: infoedit="Changes signal type without altering the binary representation.   You can changed the signal between signed and unsigned, and relocate the binary point.<br><br>Hardware notes: In hardware this block costs nothing.<br><br>Example:  Suppose the input is 6 bits wide, signed, with 2 fractional bits, and the output is forced to unsigned with 0 fractional bits.  Then an input of -2.0 (1110.00 in binary 2's complement) becomes an output of 56 (111000 in binary)."
      reinterpret2 settings: infoedit="Changes signal type without altering the binary representation.   You can changed the signal between signed and unsigned, and relocate the binary point.<br><br>Hardware notes: In hardware this block costs nothing.<br><br>Example:  Suppose the input is 6 bits wide, signed, with 2 fractional bits, and the output is forced to unsigned with 0 fractional bits.  Then an input of -2.0 (1110.00 in binary 2's complement) becomes an output of 56 (111000 in binary)."
  bus_out : Outport
  wires:
  reinterpret16/1 -> concatenate/16
  in16/1 -> reinterpret16/1
  reinterpret15/1 -> concatenate/15
  in15/1 -> reinterpret15/1
  reinterpret14/1 -> concatenate/14
  in14/1 -> reinterpret14/1
  reinterpret13/1 -> concatenate/13
  in13/1 -> reinterpret13/1
  reinterpret12/1 -> concatenate/12
  in12/1 -> reinterpret12/1
  reinterpret11/1 -> concatenate/11
  in11/1 -> reinterpret11/1
  reinterpret10/1 -> concatenate/10
  in10/1 -> reinterpret10/1
  reinterpret9/1 -> concatenate/9
  in9/1 -> reinterpret9/1
  reinterpret8/1 -> concatenate/8
  in8/1 -> reinterpret8/1
  reinterpret7/1 -> concatenate/7
  in7/1 -> reinterpret7/1
  reinterpret6/1 -> concatenate/6
  in6/1 -> reinterpret6/1
  reinterpret5/1 -> concatenate/5
  in5/1 -> reinterpret5/1
  reinterpret4/1 -> concatenate/4
  in4/1 -> reinterpret4/1
  reinterpret3/1 -> concatenate/3
  in3/1 -> reinterpret3/1
  reinterpret2/1 -> concatenate/2
  in2/1 -> reinterpret2/1
  reinterpret1/1 -> concatenate/1
  in1/1 -> reinterpret1/1
  concatenate/1 -> bus_out/1

== system snb_bc/pfb_fft/pfb_fir_generic/pfb_fir_taps/en_replicate2/bussify ==
  in1 : Inport
  in2 : Inport  Port=2
  concatenate : xbsIndex_r4/Concat  num_inputs=2  dbl_ovrd=off  block_type=concat
  reinterpret1 : xbsIndex_r4/Reinterpret  force_arith_type=on  arith_type=Unsigned  force_bin_pt=on  bin_pt=0  block_type=reinterpret
      settings: infoedit="Changes signal type without altering the binary representation.   You can changed the signal between signed and unsigned, and relocate the binary point.<br><br>Hardware notes: In hardware this block costs nothing.<br><br>Example:  Suppose the input is 6 bits wide, signed, with 2 fractional bits, and the output is forced to unsigned with 0 fractional bits.  Then an input of -2.0 (1110.00 in binary 2's complement) becomes an output of 56 (111000 in binary)."
  reinterpret2 : xbsIndex_r4/Reinterpret  force_arith_type=on  arith_type=Unsigned  force_bin_pt=on  bin_pt=0  block_type=reinterpret
      settings: infoedit="Changes signal type without altering the binary representation.   You can changed the signal between signed and unsigned, and relocate the binary point.<br><br>Hardware notes: In hardware this block costs nothing.<br><br>Example:  Suppose the input is 6 bits wide, signed, with 2 fractional bits, and the output is forced to unsigned with 0 fractional bits.  Then an input of -2.0 (1110.00 in binary 2's complement) becomes an output of 56 (111000 in binary)."
  bus_out : Outport
  wires:
  concatenate/1 -> bus_out/1
  in1/1 -> reinterpret1/1
  reinterpret1/1 -> concatenate/1
  in2/1 -> reinterpret2/1
  reinterpret2/1 -> concatenate/2

== system snb_bc/quant0/bus_mult/mult1/a_replicate/bussify ==
  in1 : Inport
  in2 : Inport  Port=2
  concatenate : xbsIndex_r4/Concat  num_inputs=2  dbl_ovrd=off  block_type=concat
  reinterpret1 : xbsIndex_r4/Reinterpret  force_arith_type=on  arith_type=Unsigned  force_bin_pt=on  bin_pt=0  block_type=reinterpret
      settings: infoedit="Changes signal type without altering the binary representation.   You can changed the signal between signed and unsigned, and relocate the binary point.<br><br>Hardware notes: In hardware this block costs nothing.<br><br>Example:  Suppose the input is 6 bits wide, signed, with 2 fractional bits, and the output is forced to unsigned with 0 fractional bits.  Then an input of -2.0 (1110.00 in binary 2's complement) becomes an output of 56 (111000 in binary)."
  reinterpret2 : xbsIndex_r4/Reinterpret  force_arith_type=on  arith_type=Unsigned  force_bin_pt=on  bin_pt=0  block_type=reinterpret
      settings: infoedit="Changes signal type without altering the binary representation.   You can changed the signal between signed and unsigned, and relocate the binary point.<br><br>Hardware notes: In hardware this block costs nothing.<br><br>Example:  Suppose the input is 6 bits wide, signed, with 2 fractional bits, and the output is forced to unsigned with 0 fractional bits.  Then an input of -2.0 (1110.00 in binary 2's complement) becomes an output of 56 (111000 in binary)."
  bus_out : Outport
  wires:
  concatenate/1 -> bus_out/1
  in1/1 -> reinterpret1/1
  reinterpret1/1 -> concatenate/1
  in2/1 -> reinterpret2/1
  reinterpret2/1 -> concatenate/2

== system snb_bc/quant0/bus_mult/mult1/b_replicate/bussify ==
  in1 : Inport
  in2 : Inport  Port=2
  concatenate : xbsIndex_r4/Concat  num_inputs=2  dbl_ovrd=off  block_type=concat
  reinterpret1 : xbsIndex_r4/Reinterpret  force_arith_type=on  arith_type=Unsigned  force_bin_pt=on  bin_pt=0  block_type=reinterpret
      settings: infoedit="Changes signal type without altering the binary representation.   You can changed the signal between signed and unsigned, and relocate the binary point.<br><br>Hardware notes: In hardware this block costs nothing.<br><br>Example:  Suppose the input is 6 bits wide, signed, with 2 fractional bits, and the output is forced to unsigned with 0 fractional bits.  Then an input of -2.0 (1110.00 in binary 2's complement) becomes an output of 56 (111000 in binary)."
  reinterpret2 : xbsIndex_r4/Reinterpret  force_arith_type=on  arith_type=Unsigned  force_bin_pt=on  bin_pt=0  block_type=reinterpret
      settings: infoedit="Changes signal type without altering the binary representation.   You can changed the signal between signed and unsigned, and relocate the binary point.<br><br>Hardware notes: In hardware this block costs nothing.<br><br>Example:  Suppose the input is 6 bits wide, signed, with 2 fractional bits, and the output is forced to unsigned with 0 fractional bits.  Then an input of -2.0 (1110.00 in binary 2's complement) becomes an output of 56 (111000 in binary)."
  bus_out : Outport
  wires:
  concatenate/1 -> bus_out/1
  in1/1 -> reinterpret1/1
  reinterpret1/1 -> concatenate/1
  in2/1 -> reinterpret2/1
  reinterpret2/1 -> concatenate/2

== system snb_bc/quant1/bus_mult/mult1/a_replicate/bussify ==
  in1 : Inport
  in2 : Inport  Port=2
  concatenate : xbsIndex_r4/Concat  num_inputs=2  dbl_ovrd=off  block_type=concat
  reinterpret1 : xbsIndex_r4/Reinterpret  force_arith_type=on  arith_type=Unsigned  force_bin_pt=on  bin_pt=0  block_type=reinterpret
      settings: infoedit="Changes signal type without altering the binary representation.   You can changed the signal between signed and unsigned, and relocate the binary point.<br><br>Hardware notes: In hardware this block costs nothing.<br><br>Example:  Suppose the input is 6 bits wide, signed, with 2 fractional bits, and the output is forced to unsigned with 0 fractional bits.  Then an input of -2.0 (1110.00 in binary 2's complement) becomes an output of 56 (111000 in binary)."
  reinterpret2 : xbsIndex_r4/Reinterpret  force_arith_type=on  arith_type=Unsigned  force_bin_pt=on  bin_pt=0  block_type=reinterpret
      settings: infoedit="Changes signal type without altering the binary representation.   You can changed the signal between signed and unsigned, and relocate the binary point.<br><br>Hardware notes: In hardware this block costs nothing.<br><br>Example:  Suppose the input is 6 bits wide, signed, with 2 fractional bits, and the output is forced to unsigned with 0 fractional bits.  Then an input of -2.0 (1110.00 in binary 2's complement) becomes an output of 56 (111000 in binary)."
  bus_out : Outport
  wires:
  reinterpret2/1 -> concatenate/2
  in2/1 -> reinterpret2/1
  reinterpret1/1 -> concatenate/1
  in1/1 -> reinterpret1/1
  concatenate/1 -> bus_out/1

== system snb_bc/quant1/bus_mult/mult1/b_replicate/bussify ==
  in1 : Inport
  in2 : Inport  Port=2
  concatenate : xbsIndex_r4/Concat  num_inputs=2  dbl_ovrd=off  block_type=concat
  reinterpret1 : xbsIndex_r4/Reinterpret  force_arith_type=on  arith_type=Unsigned  force_bin_pt=on  bin_pt=0  block_type=reinterpret
      settings: infoedit="Changes signal type without altering the binary representation.   You can changed the signal between signed and unsigned, and relocate the binary point.<br><br>Hardware notes: In hardware this block costs nothing.<br><br>Example:  Suppose the input is 6 bits wide, signed, with 2 fractional bits, and the output is forced to unsigned with 0 fractional bits.  Then an input of -2.0 (1110.00 in binary 2's complement) becomes an output of 56 (111000 in binary)."
  reinterpret2 : xbsIndex_r4/Reinterpret  force_arith_type=on  arith_type=Unsigned  force_bin_pt=on  bin_pt=0  block_type=reinterpret
      settings: infoedit="Changes signal type without altering the binary representation.   You can changed the signal between signed and unsigned, and relocate the binary point.<br><br>Hardware notes: In hardware this block costs nothing.<br><br>Example:  Suppose the input is 6 bits wide, signed, with 2 fractional bits, and the output is forced to unsigned with 0 fractional bits.  Then an input of -2.0 (1110.00 in binary 2's complement) becomes an output of 56 (111000 in binary)."
  bus_out : Outport
  wires:
  reinterpret2/1 -> concatenate/2
  in2/1 -> reinterpret2/1
  reinterpret1/1 -> concatenate/1
  in1/1 -> reinterpret1/1
  concatenate/1 -> bus_out/1

== system snb_bc/snapcoarse_0/ss/bram/mem/calc_add ==
  note: If reading/writing words
      | smaller than 32 bits,
      | change address so
      | that addressing is
      | big endian instead of
      | little, otherwise
      | pass through
  note: Use behavioural HDL
      | so that gets optimised
      | to minimum logic
  in : Inport
  add_sub : xbsIndex_r4/AddSub  mode=Subtraction  use_carryin=off  use_carryout=off  en=off  latency=0  precision=User Defined  arith_type=Unsigned  n_bits=max(1, log2(32/data_width))  bin_pt=0  quantization=Truncate  overflow=Wrap  dbl_ovrd=off  use_behavioral_HDL=on  hw_selection=Fabric  pipelined=off  block_type=addsub
  concat : xbsIndex_r4/Concat  num_inputs=2  dbl_ovrd=off  block_type=concat
  const : xbsIndex_r4/Constant  const=max(0, 32/data_width-1)  gui_display_data_type=Fixed-point  arith_type=Unsigned  n_bits=max(1, log2(32/data_width))  bin_pt=0  preci_type=Single  exp_width=8  frac_width=24  explicit_period=on  period=sample_rate  equ=P=C  opselect=C  inp2=PCIN>>17  opr=+  inp1=P  carry=CIN  dbl_ovrd=off  block_type=constant
      settings: block_version=11.4
  convert_addr : xbsIndex_r4/Convert  gui_display_data_type=Fixed-point  arith_type=Unsigned  n_bits=addr_width  bin_pt=0  float_type=Single  exp_bits=8  fraction_bits=24  quantization=Truncate  overflow=Wrap  en=off  latency=0  dbl_ovrd=off  pipeline=off  block_type=convert
      settings: xl_area=[0, 0, 0, 0, 0, 0, 0]
  lsw : xbsIndex_r4/Slice  nbits=max(1, log2(32/data_width))  boolean_output=off  mode=Lower Bit Location + Width  bit1=0  base1=MSB of Input  bit0=0  base0=LSB of Input  dbl_ovrd=off  block_type=slice
  manipulate : xbsIndex_r4/Constant  const=min(1, floor(32/data_width) - 1)  gui_display_data_type=Fixed-point  arith_type=Unsigned  n_bits=1  bin_pt=0  preci_type=Single  exp_width=8  frac_width=24  explicit_period=on  period=sample_rate  equ=P=C  opselect=C  inp2=PCIN>>17  opr=+  inp1=P  carry=CIN  dbl_ovrd=off  block_type=constant
      settings: block_version=11.4
  msw : xbsIndex_r4/Slice  nbits=addr_width - max(1, log2(32/data_width))  boolean_output=off  mode=Upper Bit Location + Width  bit1=0  base1=MSB of Input  bit0=0  base0=LSB of Input  dbl_ovrd=off  block_type=slice
  mux : xbsIndex_r4/Mux  inputs=2  en=off  latency=0  precision=Full  arith_type=Unsigned  n_bits=16  bin_pt=14  quantization=Truncate  overflow=Wrap  dbl_ovrd=off  block_type=mux
      settings: block_version=11.4
  out : Outport
  wires:
  in/1 -> convert_addr/1
  add_sub/1 -> concat/2
  msw/1 -> concat/1
  concat/1 -> mux/3
  manipulate/1 -> mux/1
  mux/1 -> out/1
  lsw/1 -> add_sub/2
  const/1 -> add_sub/1
  convert_addr/1 -> lsw/1, msw/1, mux/2
